simulink model "FilterReplay"  (R2021b)
settings: Solver=FixedStepAuto  StartTime=0.0  StopTime=900  FixedStep=0.02  RelTol=1e-3
PostLoadFcn:
  | setenv('MW_MINGW64_LOC','D:\03software\x86_64-8.1.0-release-win32-seh-rt_v6-rev0\mingw64')
settings Model: PauseTimes=0.1  Creator=kaifengqu  LastModifiedBy=KaifengQu

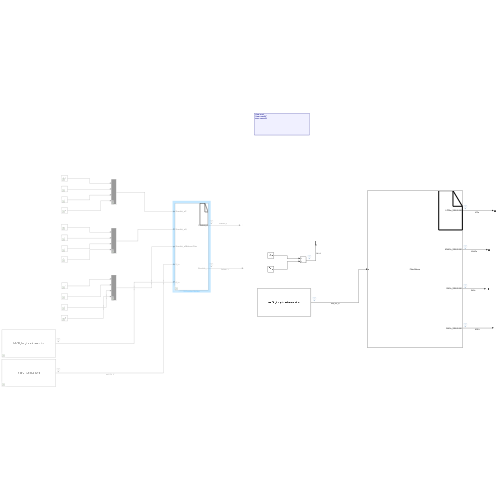
[thumbnail: Simulink's stored preview of the top-level diagram]
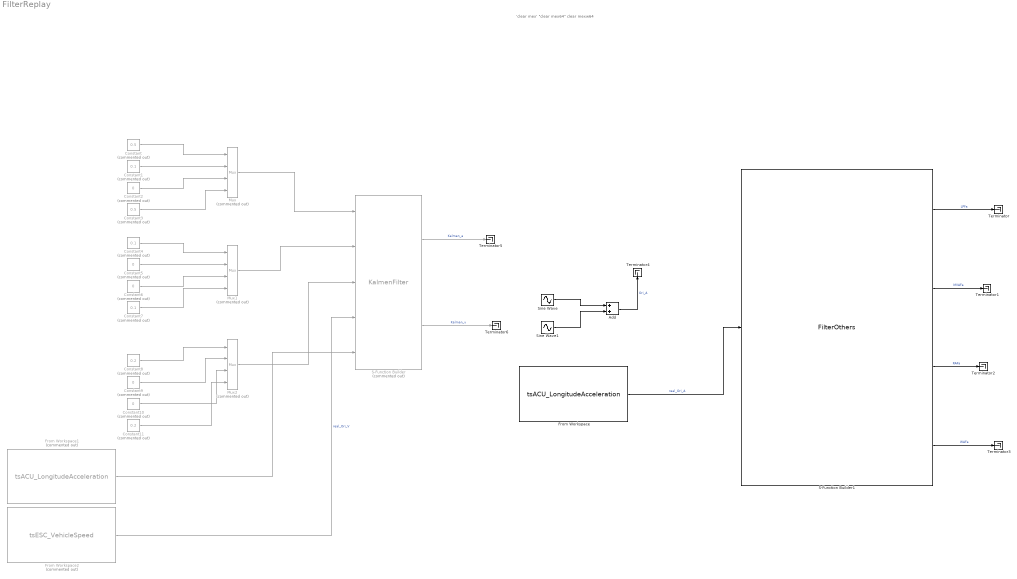
== system FilterReplay ==
  note: 'clear mex'
      | "clear mex64"
      | clear mexw64
  Add : Sum
  Constant : Constant  Commented=on  Value=0.5
  Constant1 : Constant  Commented=on  Value=0.1
  Constant{2,5..6,9..10} (5 alike) : Constant  Commented=on  Value=0
  Constant11 : Constant  Commented=on  Value=0.2
  Constant3 : Constant  Commented=on  Value=0.5
  Constant4 : Constant  Commented=on  Value=0.1
  Constant7 : Constant  Commented=on  Value=0.1
  Constant8 : Constant  Commented=on  Value=0.2
  From Workspace : FromWorkspace  VariableName=tsACU_LongitudeAcceleration
  From Workspace1 : FromWorkspace  Commented=on  VariableName=tsACU_LongitudeAcceleration
  From Workspace2 : FromWorkspace  Commented=on  VariableName=tsESC_VehicleSpeed
  Mux : Mux  Commented=on
  Mux1 : Mux  Commented=on
  Mux2 : Mux  Commented=on
  S-Function Builder : S-Function  Commented=on  FunctionName=KalmenFilter  SFunctionModules=KalmenFilter_wrapper KalmanFilter test  SFunctionDeploymentMode=off  EnableBusSupport=off  mask(S-Function Builder){}
      mask help: Simulink:masks:SFunctionBuilder_MD
      mask init:
      | val = [[.9  0.75 0.75 1 1 .9 .9 1]',[1 1 0.75 0.75 .9 .9 1 .9]'];try , sys = get_param(gcb,'SfunBuilderFcnName');if isempty(sys), sys = get_param(gcb,'FunctionName'); end,catch, sys = get_param(gcb,'FunctionName'); end
      settings: CopyFcn=set_param(gcbh,'LinkStatus','none')  OpenFcn=sfunctionwizard(gcbh)
      mask Display:
      | plot(val(:,1),val(:,2))
      | disp(sys)
      | port_label('input',1,'Simulink_aP')
      | port_label('input',2,'Simulink_aQ')
      | port_label('input',3,'Simulink_aR')
      | port_label('input',4,'V_in')
      | port_label('input',5,'A_in')
      | port_label('output',1,'Simulink_a')
      | port_label('output',2,'Simulink_v')
  S-Function Builder1 : S-Function  FunctionName=FilterOthers  SFunctionModules=FilterOthers_wrapper RecursiveAveragingFilter testMain LowerPassFilter MiddleValueAveragingFilter WeightedaveragingFilter  SFunctionDeploymentMode=off  EnableBusSupport=off  mask(S-Function Builder){}
      mask help: Simulink:masks:SFunctionBuilder_MD
      mask init: same as FilterReplay/S-Function Builder
      settings: CopyFcn=set_param(gcbh,'LinkStatus','none')  OpenFcn=sfunctionwizard(gcbh)
      mask Display:
      | plot(val(:,1),val(:,2))
      | disp(sys)
      | port_label('input',1,'a')
      | port_label('output',1,'LPFAa_SIMULINK')
      | port_label('output',2,'MVAFa_SIMULINK')
      | port_label('output',3,'RAFa_SIMULINK')
      | port_label('output',4,'WAFa_SIMULINK')
  Sine Wave : Sin  SampleTime=0
  Sine Wave1 : Sin  Amplitude=0.075  Frequency=50  SampleTime=0
  Terminator{,1..6} (7 alike) : Terminator
  wires:
  Constant/1 -> Mux/1
  Constant1/1 -> Mux/2
  Constant2/1 -> Mux/3
  Constant3/1 -> Mux/4
  Constant4/1 -> Mux1/1
  Constant5/1 -> Mux1/2
  Constant6/1 -> Mux1/3
  Constant7/1 -> Mux1/4
  Mux1/1 -> S-Function Builder/2
  Mux/1 -> S-Function Builder/1
  Constant8/1 -> Mux2/1
  Constant9/1 -> Mux2/2
  Constant10/1 -> Mux2/3
  Constant11/1 -> Mux2/4
  Mux2/1 -> S-Function Builder/3
  S-Function Builder/1 -> Terminator5/1  "Kalman_a"
  S-Function Builder/2 -> Terminator6/1  "Kalman_v"
  S-Function Builder1/1 -> Terminator/1  "LPFa"
  S-Function Builder1/2 -> Terminator1/1  "MVAFa"
  S-Function Builder1/3 -> Terminator2/1  "RAFa"
  S-Function Builder1/4 -> Terminator3/1  "WAFa"
  Sine Wave/1 -> Add/1
  Sine Wave1/1 -> Add/2
  Add/1 -> Terminator4/1  "Ori_A"
  From Workspace/1 -> S-Function Builder1/1  "real_Ori_A"
  From Workspace1/1 -> S-Function Builder/5
  From Workspace2/1 -> S-Function Builder/4  "real_Ori_V"
